simulink model "GSK_PVModel_01"  (R2016a)
settings: Solver=ode2  StartTime=0.0  StopTime=10.0  RelTol=1e-3
values from neighbouring files (symbols this model uses):
  a = 1.5    [GSK_PVModelValues.m]    (also in GSK_PVModelValues_05.m)
  G_n = 1000    [GSK_PVModelValues.m]    (also in GSK_PVModelValues_05.m)
  I_pv_n = 6.5    [GSK_PVModelValues.m]    (also in GSK_PVModelValues_05.m)
  I_sc_n = 6.43    [GSK_PVModelValues.m]    (also in GSK_PVModelValues_05.m)
  k = physconst('Boltzmann')    [GSK_PVModelValues.m]    (also in GSK_PVModelValues_05.m)
  K_I = 3.5e-3    (= 0.0035)    [GSK_PVModelValues.m]    (also in GSK_PVModelValues_05.m)
  K_V = - 235.5e-3    (= -0.2355)    [GSK_PVModelValues.m]    (also in GSK_PVModelValues_05.m)
  N_s = 128    [GSK_PVModelValues.m]    (also in GSK_PVModelValues_05.m)
  q = 1.60217662e-19    [GSK_PVModelValues.m]    (also in GSK_PVModelValues_05.m)
  R_p = 1000    [GSK_PVModelValues.m]    (also in GSK_PVModelValues_05.m)
  R_s = 1e-3    (= 0.001)    [GSK_PVModelValues.m]    (also in GSK_PVModelValues_05.m = 0.128)
  T = 273+40    (= 313)    [GSK_PVModelValues.m]    (also in GSK_PVModelValues_05.m)
  T_n = 25+273    (= 298)    [GSK_PVModelValues.m]    (also in GSK_PVModelValues_05.m)
  V_oc_n = 85.6    [GSK_PVModelValues.m]    (also in GSK_PVModelValues_05.m)
libraries: fl_lib x14, nesl_utility x4, simulink x2, powerlib_meascontrol x1
settings Model: Creator=gadis  LastModifiedBy=gadis

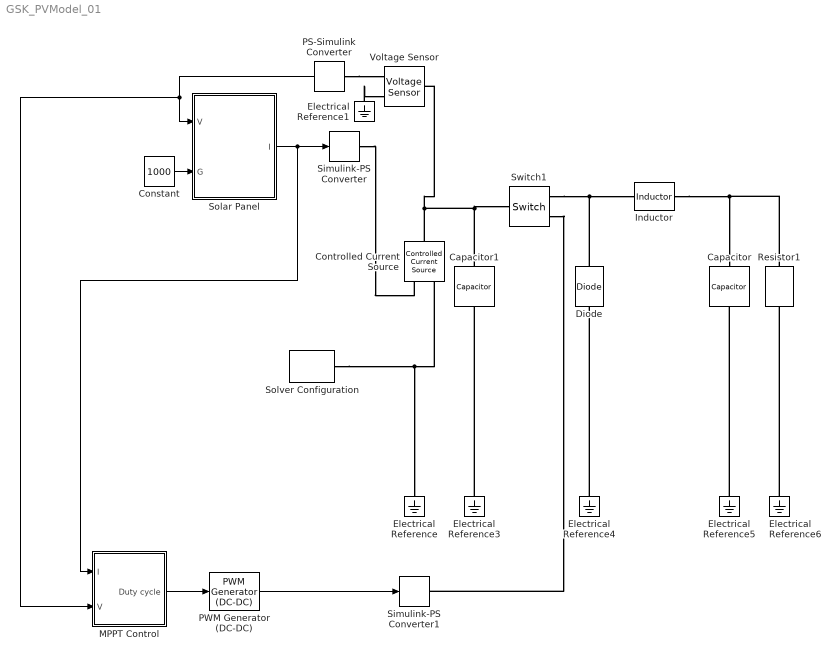
== system GSK_PVModel_01 ==
  Capacitor : fl_lib/Electrical/Electrical Elements/Capacitor  c=0.5 mF  r=1e-6 Ohm  g=0 1/Ohm  i_specify=off  i_priority=None  i=0 A  v_specify=off  v_priority=None  v=0 V  vc_specify=off  vc_priority=High  vc=0 V
  Capacitor1 : fl_lib/Electrical/Electrical Elements/Capacitor  c=0.5 mF  r=1e-6 Ohm  g=0 1/Ohm  i_specify=off  i_priority=None  i=0 A  v_specify=off  v_priority=None  v=0 V  vc_specify=off  vc_priority=High  vc=0 V
  Constant : Constant  Value=1000
  Controlled Current Source : fl_lib/Electrical/Electrical Sources/Controlled Current Source
  Diode : fl_lib/Electrical/Electrical Elements/Diode  Vf=0.6 V  Ron=0.3 Ohm  Goff=1e-8 1/Ohm  i_specify=off  i_priority=None  i=0 A  v_specify=off  v_priority=None  v=0 V
  Electrical Reference{,1,3..6} (6 alike) : fl_lib/Electrical/Electrical Elements/Electrical Reference
  Inductor : fl_lib/Electrical/Electrical Elements/Inductor  l=5 mH  r=0 Ohm  g=1e-9 1/Ohm  i_specify=off  i_priority=None  i=0 A  v_specify=off  v_priority=None  v=0 V  i_L_specify=off  i_L_priority=High  i_L=0 A
  MPPT Control : Subsystem
  PS-Simulink Converter : nesl_utility/PS-Simulink Converter  PhysicalDomain=network_engine_domain  SubClassName=ps_output  LeftPortType=input  RightPortType=output  PseudoPeriodic=off  Frequencies=[]  Unit=1  AffineConversion=off
  PWM Generator (DC-DC) : powerlib_meascontrol/Pulse & Signal Generators/PWM Generator (DC-DC)  Fsw=60000  Ts=0
  Resistor1 : fl_lib/Electrical/Electrical Elements/Resistor  R=1 Ohm  i_specify=off  i_priority=None  i=0 A  v_specify=off  v_priority=None  v=0 V
  Simulink-PS Converter : nesl_utility/Simulink-PS Converter  PhysicalDomain=network_engine_domain  SubClassName=ps_input  LeftPortType=input  RightPortType=output  PseudoPeriodic=off  Frequencies=[]  NoiseDistribution=none  NoiseParameters=[]  Unit=1  AffineConversion=off  InputFiltering=off  SimscapeFilterOrder=1  InputFilterTimeConstant=0.001  UdotUserProvided=1
  Simulink-PS Converter1 : nesl_utility/Simulink-PS Converter  PhysicalDomain=network_engine_domain  SubClassName=ps_input  LeftPortType=input  RightPortType=output  PseudoPeriodic=off  Frequencies=[]  NoiseDistribution=none  NoiseParameters=[]  Unit=1  AffineConversion=off  InputFiltering=off  SimscapeFilterOrder=1  InputFilterTimeConstant=0.001  UdotUserProvided=1
  Solar Panel : Subsystem
  Solver Configuration : nesl_utility/Solver Configuration  PhysicalDomain=network_engine_domain  SubClassName=solver  LeftPortType=input  RightPortType=generic  Accelerate=off  Tones=[]  Harmonics=[]  SimulateNoise=off  Profile=off  UseLocalSampling=off  EnableSwitchedLinearOptims=on  FrequencyDomain=off  UseCCode=off  RelTol=0.001  AbsTol=1e-06  MinStep=1e-09  ToWorkspace=off  RevertToSquareIcSolve=off  NumHomotopyIterations=100  PhasorMode=off  PhasorModeNumHarmonics=1  OverrideAbsTol=off  DoDC=off  ResidualTolerance=1e-09  UseLocalSolver=off  LocalSolverChoice=NE_BACKWARD_EULER_ADVANCER  LocalSolverSampleTime=0.001  DoFixedCost=off  MaxNonlinIter=3  MaxModeIter=2  LinearAlgebra=Sparse  DelaysMemoryBudget=1024  AutomaticFiltering=on  FilteringTimeConstant=0.001
  Switch1 : fl_lib/Electrical/Electrical Elements/Switch  R_closed=0.001 Ohm  G_open=1e-8 1/Ohm  Threshold=0  i_specify=off  i_priority=None  i=0 A  v_specify=off  v_priority=None  v=0 V
  Voltage Sensor : fl_lib/Electrical/Electrical Sensors/Voltage Sensor
  wires:
  PS-Simulink Converter/1 -> MPPT Control/2(V), Solar Panel/1(V)
  Constant/1 -> Solar Panel/2(G)
  PWM Generator (DC-DC)/1 -> Simulink-PS Converter1/1
  MPPT Control/1(Duty cycle) -> PWM Generator (DC-DC)/1
  Solar Panel/1(I) -> MPPT Control/1(I), Simulink-PS Converter/1
  connections:
  Simulink-PS Converter/RConn1 -- Controlled Current Source/RConn1
  Electrical Reference1/LConn1 -- Voltage Sensor/RConn2
  PS-Simulink Converter/LConn1 -- Voltage Sensor/RConn1
  Inductor/RConn1 -- Resistor1/LConn1 -- Capacitor/LConn1
  Diode/RConn1 -- Switch1/RConn2 -- Inductor/LConn1
  Capacitor1/LConn1 -- Controlled Current Source/LConn1 -- Voltage Sensor/LConn1 -- Switch1/LConn1
  Electrical Reference3/LConn1 -- Capacitor1/RConn1
  Electrical Reference4/LConn1 -- Diode/LConn1
  Switch1/RConn1 -- Simulink-PS Converter1/RConn1
  Electrical Reference5/LConn1 -- Capacitor/RConn1
  Electrical Reference6/LConn1 -- Resistor1/RConn1
  Solver Configuration/RConn1 -- Electrical Reference/LConn1 -- Controlled Current Source/RConn2

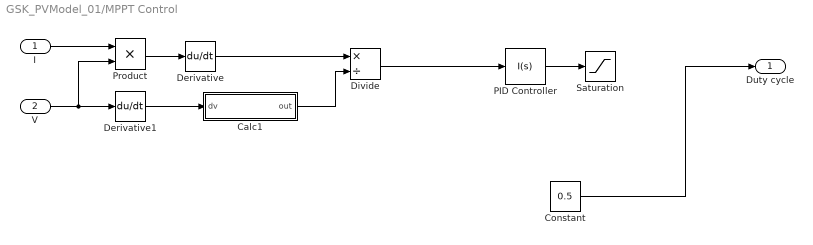
== system GSK_PVModel_01/MPPT Control ==
  I : Inport
  V : Inport  Port=2
  Calc1 : MATLAB Function  TreatAsAtomicUnit=on
  Constant : Constant  Value=0.5
  Derivative : Derivative
  Derivative1 : Derivative
  Divide : Product  Inputs=*/
  PID Controller : simulink/Continuous/PID Controller  Controller=I  TimeDomain=Continuous-time  SampleTime=-1  IntegratorMethod=Forward Euler  FilterMethod=Forward Euler  Form=Parallel  UseFilter=on  ControllerParametersSource=internal  P=0.001  I=0.001  D=0  N=100  InitialConditionSource=internal  InitialConditionForIntegrator=0  InitialConditionForFilter=0  ExternalReset=none  LimitOutput=off  UpperSaturationLimit=inf  LowerSaturationLimit=-inf  LinearizeAsGain=on  AntiWindupMode=none  Kb=1  TrackingMode=off  Kt=1  PParamMin=[]  PParamMax=[]  IParamMin=[]  IParamMax=[]  DParamMin=[]  DParamMax=[]  NParamMin=[]  NParamMax=[]  KbParamMin=[]  KbParamMax=[]  KtParamMin=[]  KtParamMax=[]  POutMin=[]  POutMax=[]  IOutMin=[]  IOutMax=[]  DOutMin=[]  DOutMax=[]  NOutMin=[]  NOutMax=[]  KbOutMin=[]  KbOutMax=[]  KtOutMin=[]  KtOutMax=[]  IntegratorOutMin=[]  IntegratorOutMax=[]  FilterOutMin=[]  FilterOutMax=[]  SumOutMin=[]  SumOutMax=[]  SumI1OutMin=[]  SumI1OutMax=[]  SumI2OutMin=[]  SumI2OutMax=[]  SumI3OutMin=[]  SumI3OutMax=[]  SumDOutMin=[]  SumDOutMax=[]  SaturationOutMin=[]  SaturationOutMax=[]  IntegratorContinuousStateAttributes=''  IntegratorStateMustResolveToSignalObject=off  IntegratorRTWStateStorageClass=Auto  FilterContinuousStateAttributes=''  FilterStateMustResolveToSignalObject=off  FilterRTWStateStorageClass=Auto  DifferentiatorICPrevScaledInput=0  DifferentiatorOutMin=[]  DifferentiatorOutMax=[]
  Product : Product
  Saturation : Saturate  UpperLimit=1  LowerLimit=0
  Duty cycle : Outport
  wires:
  I/1 -> Product/1
  V/1 -> Derivative1/1, Product/2
  Product/1 -> Derivative/1
  Derivative/1 -> Divide/1
  Derivative1/1 -> Calc1/1(dv)
  PID Controller/1 -> Saturation/1
  Calc1/1(out) -> Divide/2
  Divide/1 -> PID Controller/1
  Constant/1 -> Duty cycle/1

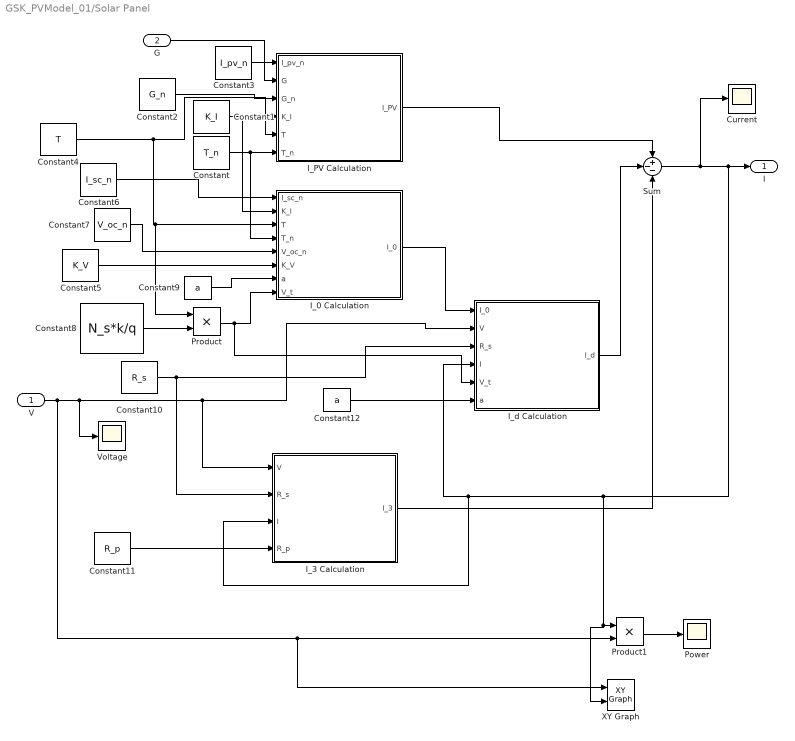
== system GSK_PVModel_01/Solar Panel ==
  V : Inport
  G : Inport  Port=2
  Constant : Constant  Value=T_n
  Constant1 : Constant  Value=K_I
  Constant10 : Constant  Value=R_s
  Constant11 : Constant  Value=R_p
  Constant12 : Constant  Value=a
  Constant2 : Constant  Value=G_n
  Constant3 : Constant  Value=I_pv_n
  Constant4 : Constant  Value=T
  Constant5 : Constant  Value=K_V
  Constant6 : Constant  Value=I_sc_n
  Constant7 : Constant  Value=V_oc_n
  Constant8 : Constant  Value=N_s*k/q
  Constant9 : Constant  Value=a
  Current : Scope
  I_0 Calculation : MATLAB Function  TreatAsAtomicUnit=on
  I_3 Calculation : MATLAB Function  TreatAsAtomicUnit=on
  I_PV Calculation : MATLAB Function  TreatAsAtomicUnit=on
  I_d Calculation : MATLAB Function  TreatAsAtomicUnit=on
  Power : Scope
  Product : Product
  Product1 : Product
  Sum : Sum  Inputs=+--
  Voltage : Scope
  XY Graph : simulink/Sinks/XY Graph  xmin=-1  xmax=100  ymin=-1  ymax=10  st=-1
  I : Outport
  wires:
  Product/1 -> I_d Calculation/5(V_t), I_0 Calculation/8(V_t)
  Constant9/1 -> I_0 Calculation/7(a)
  Constant3/1 -> I_PV Calculation/1(I_pv_n)
  Constant/1 -> I_0 Calculation/4(T_n), I_PV Calculation/6(T_n)
  Constant5/1 -> I_0 Calculation/6(K_V)
  Constant2/1 -> I_PV Calculation/3(G_n)
  Constant1/1 -> I_0 Calculation/2(K_I), I_PV Calculation/4(K_I)
  Constant6/1 -> I_0 Calculation/1(I_sc_n)
  Constant7/1 -> I_0 Calculation/5(V_oc_n)
  Constant4/1 -> Product/1, I_0 Calculation/3(T), I_PV Calculation/5(T)
  I_0 Calculation/1(I_0) -> I_d Calculation/1(I_0)
  Constant12/1 -> I_d Calculation/6(a)
  Constant8/1 -> Product/2
  I_PV Calculation/1(I_PV) -> Sum/1
  I_d Calculation/1(I_d) -> Sum/2
  V/1 -> XY Graph/1, Product1/2, Voltage/1, I_3 Calculation/1(V), I_d Calculation/2(V)
  Sum/1 -> Current/1, XY Graph/2, Product1/1, I_3 Calculation/3(I), I_d Calculation/4(I), I/1
  Constant11/1 -> I_3 Calculation/4(R_p)
  Constant10/1 -> I_3 Calculation/2(R_s), I_d Calculation/3(R_s)
  I_3 Calculation/1(I_3) -> Sum/3
  G/1 -> I_PV Calculation/2(G)
  Product1/1 -> Power/1

== matlab function GSK_PVModel_01/Solar Panel/I_PV Calculation ==
  data: I_pv_n input; I_PV output; G input; G_n input; K_I input; T input; T_n input
function I_PV = fcn(I_pv_n, G, G_n, K_I, T, T_n )
%#codegen
Delta_T = (T - T_n);
I_PV = (I_pv_n + K_I*Delta_T)*G/G_n;

== matlab function GSK_PVModel_01/Solar Panel/I_0 Calculation ==
  data: I_sc_n input; K_I input; T input; T_n input; I_0 output; V_oc_n input; K_V input; a input; V_t input
function I_0 = fcn(I_sc_n, K_I, T, T_n, V_oc_n, K_V, a, V_t)
%#codegen
Delta_T = (T - T_n);
I_0 = (I_sc_n + K_I * Delta_T )/(exp((V_oc_n + K_V*Delta_T)/(a*V_t))-1);

== matlab function GSK_PVModel_01/Solar Panel/I_d Calculation ==
  data: I_0 input; V input; R_s input; I input; V_t input; I_d output; a input
function I_d = fcn(I_0, V, R_s, I, V_t, a)
%#codegen
I_d = I_0*(exp((V+R_s*I)/(V_t*a))-1);

== matlab function GSK_PVModel_01/Solar Panel/I_3 Calculation ==
  data: V input; R_s input; I input; R_p input; I_3 output
function I_3 = fcn(V, R_s, I, R_p)
%#codegen
I_3 = (V+R_s*I)/R_p;

== matlab function GSK_PVModel_01/MPPT Control/Calc1 ==
  data: dv input; out output
function out = fcn(dv)
%#codegen
if dv == 0
    out = 0.01;
else
    out = dv;
end
